simulink model "pseissimulink"  (R2024b)
settings: Solver=VariableStepAuto  StartTime=0.0  StopTime=0.01  MaxStep=0.001  RelTol=1e-3
InitFcn:
  | L = 0.002;
  | R = 10;
  | C = 0.00001;
  | Uin = 32;
  | d = 40000;

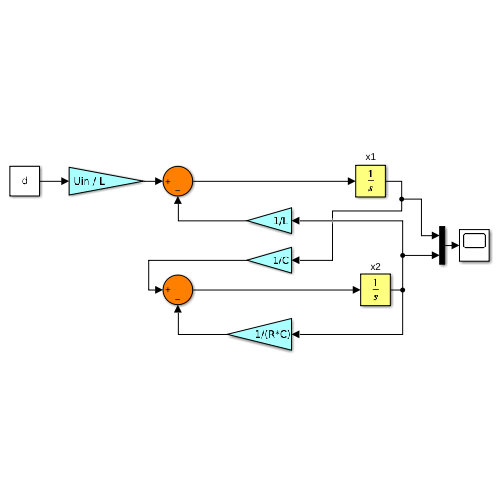
[thumbnail: Simulink's stored preview of the top-level diagram]
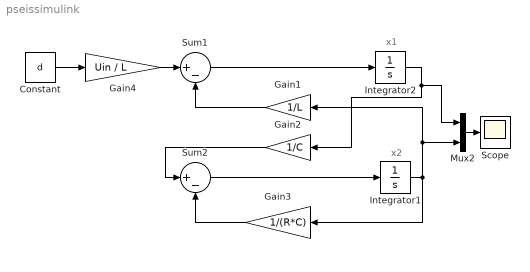
== system pseissimulink ==
  note: x1
  note: x2
  Constant : Constant  Value=d
  Gain1 : Gain  Gain=1/L
  Gain2 : Gain  Gain=1/C
  Gain3 : Gain  Gain=1/(R*C)
  Gain4 : Gain  Gain=Uin / L
  Integrator1 : Integrator
  Integrator2 : Integrator
  Mux2 : Mux  Inputs=2
  Scope : Scope
  Sum1 : Sum  Inputs=|+-
  Sum2 : Sum  Inputs=|+-
  wires:
  Sum1/1 -> Integrator2/1
  Gain1/1 -> Sum1/2
  Mux2/1 -> Scope/1
  Sum2/1 -> Integrator1/1
  Gain4/1 -> Sum1/1
  Gain2/1 -> Sum2/1
  Gain3/1 -> Sum2/2
  Integrator2/1 -> Mux2/1, Gain2/1
  Integrator1/1 -> Mux2/2, Gain1/1, Gain3/1
  Constant/1 -> Gain4/1
